simulink model "central_dynamics"  (R2023a)
settings: Solver=VariableStepAuto  StartTime=0.0  StopTime=10  RelTol=1e-3
undefined symbols (not defined in the file or in its folder): f, Payload
libraries: uavmavlinklib x3, instrumentlib x2
settings Model: Creator=Marek  LastModifiedBy=Marek

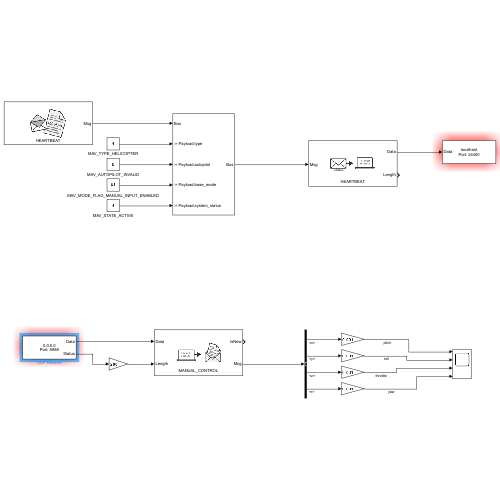
[thumbnail: Simulink's stored preview of the top-level diagram]
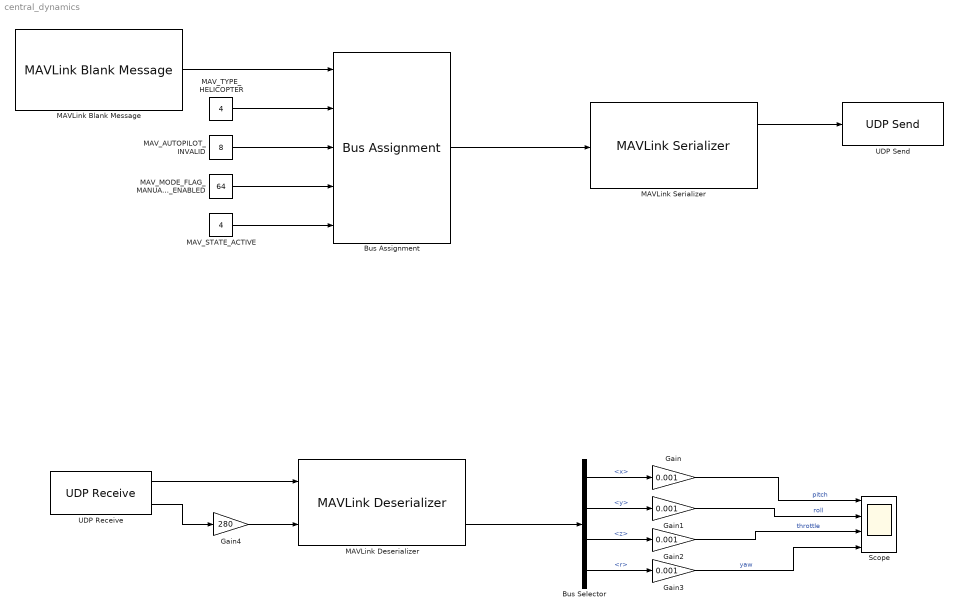
== system central_dynamics ==
  Bus Assignment : BusAssignment  AssignedSignals=Payload.type,Payload.autopilot,Payload.base_mode,Payload.system_status
  Bus Selector : BusSelector  OutputSignals=Payload.x,Payload.y,Payload.z,Payload.r
  Gain{,1..3} (4 alike) : Gain  Gain=0.001
  Gain4 : Gain  Gain=280  OutDataTypeStr=uint16
  MAVLink Blank Message : uavmavlinklib/MAVLink Blank Message  dialectSource=Select from standard MAVLink dialects  dialect=common.xml  dialectCustom=common.xml  version=2  messageType=HEARTBEAT  SystemID=1  ComponentID=26  SampleTime=[0, 1]
  MAVLink Deserializer : uavmavlinklib/MAVLink Deserializer  dialectSource=Select from standard MAVLink dialects  dialect=common.xml  dialectCustom=common.xml  version=2  messageType=MANUAL_CONTROL  inputDataLength=on  SystemIDFilter=off  systemID=1  ComponentIDFilter=off  componentID=1  queueMsg=off  queueMsgSize=50  dropNum=off
  MAVLink Serializer : uavmavlinklib/MAVLink Serializer  dialectSource=Select from standard MAVLink dialects  dialect=common.xml  dialectCustom=common.xml  version=2  messageType=HEARTBEAT
  MAV_AUTOPILOT_INVALID : Constant  Value=8  OutDataTypeStr=uint8
  MAV_MODE_FLAG_MANUAL_INPUT_ENABLED : Constant  Value=64  OutDataTypeStr=uint8
  MAV_STATE_ACTIVE : Constant  Value=4  OutDataTypeStr=uint8
  MAV_TYPE_HELICOPTER : Constant  Value=4  OutDataTypeStr=uint8
  Scope : Scope  NumInputPorts=4
  UDP Receive : instrumentlib/UDP Receive  LocalAddress=0.0.0.0  LocalPort=port_number  EnablePortSharing=off  Host=localhost  Port=24400  GetLatestData=off  DataSize=280  DataType=uint8  ASCIIFormatting=%f,  Terminator=LF  CustomTerminator=10  ByteOrder=big-endian  EnableBlockingMode=off  Timeout=10  SampleTime=0.001  SimulateUsing=Interpreted execution
  UDP Send : instrumentlib/UDP Send  Host=localhost  Port=24400  LocalAddress=0.0.0.0  LocalPort=port_number  EnablePortSharing=off  OutputDatagramPacketSize=280  ByteOrder=big-endian  EnableBlockingMode=off  SimulateUsing=Interpreted execution
  wires:
  UDP Receive/1 -> MAVLink Deserializer/1
  MAVLink Deserializer/2 -> Bus Selector/1
  Bus Selector/1 -> Gain/1  "<x>"
  Bus Selector/2 -> Gain1/1  "<y>"
  Bus Selector/3 -> Gain2/1  "<z>"
  Bus Selector/4 -> Gain3/1  "<r>"
  Gain/1 -> Scope/1  "pitch"
  Gain1/1 -> Scope/2  "roll"
  Gain2/1 -> Scope/3  "throttle"
  Gain3/1 -> Scope/4  "yaw"
  Gain4/1 -> MAVLink Deserializer/2
  UDP Receive/2 -> Gain4/1
  MAVLink Blank Message/1 -> Bus Assignment/1
  Bus Assignment/1 -> MAVLink Serializer/1
  MAVLink Serializer/1 -> UDP Send/1
  MAV_AUTOPILOT_INVALID/1 -> Bus Assignment/3
  MAV_STATE_ACTIVE/1 -> Bus Assignment/5
  MAV_MODE_FLAG_MANUAL_INPUT_ENABLED/1 -> Bus Assignment/4
  MAV_TYPE_HELICOPTER/1 -> Bus Assignment/2
